simulink model "FuzzyWuzzy"  (R2013a)
settings: Solver=FixedStepDiscrete  StartTime=0.0  StopTime=10.0  FixedStep=0.01  RelTol=1e-3
libraries: fuzblock x1
settings Model: Creator=val  LastModifiedBy=val
settings HardwareCC: ProdBitPerInt=16  ProdBitPerPointer=8  ProdIntDivRoundTo=Zero  ProdEndianess=LittleEndian  ProdWordSize=8  ProdHWDeviceType=Atmel->AVR
settings RTWCC: RTWCompilerOptimization=On

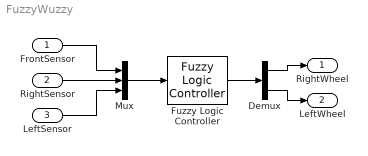
== system FuzzyWuzzy ==
  FrontSensor : Inport
  RightSensor : Inport  Port=2
  LeftSensor : Inport  Port=3
  Demux : Demux  Outputs=2
  Fuzzy Logic Controller : fuzblock/Fuzzy Logic  Controller  fis='Lab4Fuzzy.fis'
  Mux : Mux  Inputs=3
  RightWheel : Outport
  LeftWheel : Outport  Port=2
  wires:
  RightSensor/1 -> Mux/2
  FrontSensor/1 -> Mux/1
  LeftSensor/1 -> Mux/3
  Demux/2 -> LeftWheel/1
  Demux/1 -> RightWheel/1
  Fuzzy Logic Controller/1 -> Demux/1
  Mux/1 -> Fuzzy Logic Controller/1
